simulink model "PubIfDecisionTOS_MDL"  (R2020b)
settings: configuration reference "DspaceConfig" (kept outside this file)
PostLoadFcn:
  | if any(exist('dsrtsu_mdlpostloadfcn', 'file') ~= 0), dsrtsu_mdlpostloadfcn('Execute', bdroot); end
InitFcn:
  | , if any(exist('dsmpb_private', 'file') ~= 0), dsmpb_private('dsmpb_mdlclblib', 'Init', bdroot); end,
undefined symbols (not defined in the file or in its folder): C_TOS_ACCEgoRAxletoFbumplength_m, C_TOS_ACCTargetFront_Flag, C_TOS_AEBJAPedObjDxThre_Val, C_TOS_AEBJAPedObjDyThre_Val, C_TOS_AEBJATargetSize_Val, C_TOS_AEBJAVehObjDxThre_Val, C_TOS_AEBJAVehObjDyThre_Val, C_TOS_AEBJuncPedTargetSize_Val, C_TOS_AEBLatObjDxThre_Val, C_TOS_AEBLatPedDyThre_Val, C_TOS_AEBLatTargetSize_Val, C_TOS_AEBLongTargetInEgoFront_Flag, C_TOS_axAbsGround_Parameter, C_TOS_CameraConfirmedFlag, C_TOS_CNsubjWidth, C_TOS_CurrentLaneCoreMinWidth_Val, C_TOS_CutInProb_Val_Zero, C_TOS_CutOutProb_Val_Zero, C_TOS_D2R_Val, C_TOS_DefaultValueObjectToCenterLine_dy, C_TOS_EgoCarWidth_Val, C_TOS_EgoDxRefPoint_m, C_TOS_EgoRAxletoFbumplength_m, C_TOS_HalfWidthVehicle_Con, C_TOS_HWA_CurrentLaneFlag, C_TOS_HWA_LeftLaneFlag, C_TOS_HWA_MovingDir_Vaild, C_TOS_HWA_MovState_Vaild, C_TOS_HWA_RightLaneFlag, C_TOS_LaneLineCourseErrorFront, C_TOS_LaneLineCourseErrorRear, C_TOS_MotorbikeDefaultWidth_m, C_TOS_NumberOfEffectiveTargets, C_TOS_Obj_Age_Val, C_TOS_Objdx_Constraint_Val, C_TOS_ObjectDefaultWidth_m, C_TOS_ObjInCurrentLane_Val, C_TOS_ObjInCurrentLaneValid, C_TOS_ObjInLeftLaneValid, C_TOS_ObjInRightLaneValid, C_TOS_ObjNotInCurrentLane_Val, C_TOS_ObjNotREElementType, C_TOS_ObjPredictDis_dy_ConstantVal_Zeros, C_TOS_ObjToCenterLine_ConstantVal_Zeros, C_TOS_OFMObjIDInvilad_Val, C_TOS_PIL_LatDisCons_Val_zero, C_TOS_PIL_ObjectCutInFlag_b, C_TOS_PIL_ObjectCutOutFlag_b, C_TOS_PIL_ObjLaneProb_al_Val, C_TOS_PP_ObjFusType_FC_Confirm_b, C_TOS_PP_ObjFusType_FC_FR_Confirm_b, C_TOS_PP_ObjFusType_FR_Confirm_b, C_TOS_RE_80BoolDefault_Val, C_TOS_RE_80Single181Default_Val, C_TOS_RE_80Single255Default_Val, C_TOS_RE_80Uint8Default_Val, C_TOS_RE_D2R, C_TOS_RE_D_180_Val, C_TOS_RE_InvalidObjectID_Val, C_TOS_RE_InvalidTargetChainDir_Val ... (+142)
libraries: simulink x1650, TOS_LIB x361, canfdmsglib x14
(part 47 of 69)

== system PubIfDecisionTOS_MDL/TOS_20201112/TOS_2012080320/TOS/AEB/TOS_AEBJunct_20201208/AEBJunc_Object_Condition1/AEBJA_TargetCondition/TOS_AEBJunc_TargetsCondition/AEBJunc_VehTargetCondition/AEBJunc_VehTargetObjectTypeFlag ==
  ObjectType : Inport
  AEBJunc_VehTarget_ID_K1 : Inport  Port=2
  ObjectID : Inport  Port=3
  AEBJunc_VehTargetObjectTypeAborDly : Subsystem
  Compare To Constant3 : simulink/Logic and Bit Operations/Compare To Constant  relop===  const=OFM_OBJ_TYPE_E.CAR  OutDataTypeStr=boolean
      settings: AttributesFormatString=%<const>
  Compare To Constant4 : simulink/Logic and Bit Operations/Compare To Constant  relop===  const=OFM_OBJ_TYPE_E.TRUCK  OutDataTypeStr=boolean
      settings: AttributesFormatString=%<const>
  Data Type Conversion : DataTypeConversion  OutDataTypeStr=Enum: OFM_OBJ_TYPE_E
  Logical Operator3 : Logic  Operator=OR  AllPortsSameDT=off  OutDataTypeStr=boolean
  AEBJunc_VehTargetObjectTypeFlag : Outport
  wires:
  AEBJunc_VehTargetObjectTypeAborDly/1(TOS_AEBJunc_VehObjectTypeFilt) -> AEBJunc_VehTargetObjectTypeFlag/1
  ObjectID/1 -> AEBJunc_VehTargetObjectTypeAborDly/2(ObjectID)
  AEBJunc_VehTarget_ID_K1/1 -> AEBJunc_VehTargetObjectTypeAborDly/1(AEBJunc_VehTarget_ID_K1)
  Compare To Constant4/1 -> Logical Operator3/2
  Compare To Constant3/1 -> Logical Operator3/1
  Data Type Conversion/1 -> Compare To Constant4/1, Compare To Constant3/1
  ObjectType/1 -> Data Type Conversion/1
  Logical Operator3/1 -> AEBJunc_VehTargetObjectTypeAborDly/3(TOS_AEBJunc_VehObjectType)

== system PubIfDecisionTOS_MDL/TOS_20201112/TOS_2012080320/TOS/AEB/TOS_AEBJunct_20201208/AEBJunc_Object_Condition1/AEBJA_TargetCondition/TOS_AEBJunc_TargetsCondition/AEBJunc_VehTargetCondition/Subsystem ==
  Object_MovingState : Inport
  Compare To Constant1 : simulink/Logic and Bit Operations/Compare To Constant  relop===  const=OFM_OBJ_MOVINGSTATE_E.MOVING  OutDataTypeStr=boolean
      settings: AttributesFormatString=%<const> = 2
  Compare To Constant2 : simulink/Logic and Bit Operations/Compare To Constant  relop===  const=OFM_OBJ_MOVINGSTATE_E.MOVING_SLOWLY  OutDataTypeStr=boolean
      settings: AttributesFormatString=%<const> = 5
  Data Type Conversion : DataTypeConversion  OutDataTypeStr=Enum: OFM_OBJ_MOVINGSTATE_E
  Logical Operator1 : Logic  Operator=OR  AllPortsSameDT=off  OutDataTypeStr=boolean
  TOS_AEBJuncVehTargetMovStateFlg : Outport
  wires:
  Data Type Conversion/1 -> Compare To Constant1/1, Compare To Constant2/1
  Object_MovingState/1 -> Data Type Conversion/1
  Compare To Constant2/1 -> Logical Operator1/2
  Logical Operator1/1 -> TOS_AEBJuncVehTargetMovStateFlg/1
  Compare To Constant1/1 -> Logical Operator1/1

== system PubIfDecisionTOS_MDL/TOS_20201112/TOS_2012080320/TOS/AEB/TOS_AEBJunct_20201208/AEBJunc_Object_Condition1/AEBJA_TargetCondition/TOS_AEBJunc_TargetsCondition/AEBJunc_VehTargetCondition/TOS_AEBJunc_VehTargetMoveDir ==
  Object_Dx : Inport
  PP_ObjMovingDirSignalProcessing : Inport  Port=2
  Object_HeadingAngle : Inport  Port=3
  Object_VX : Inport  Port=4
  Object_VY : Inport  Port=5
  VIE_EgoVelocity : Inport  Port=6
  axvRefMs2 : Inport  Port=7
  Abs{,1..3} (4 alike) : Abs
  Add{,2..4} (4 alike) : Sum
  Add1 : Sum  Inputs=+-
  Compare To Constant : simulink/Logic and Bit Operations/Compare To Constant  relop=<  const=P_TOS_OncomingTarget_VxabsOffset_val  OutDataTypeStr=boolean
      settings: AttributesFormatString=%<const> = -0.7m/s
  Compare To Constant1 : simulink/Logic and Bit Operations/Compare To Constant  relop=>  const=P_TOS_CrossingTargetVyvThre_val  OutDataTypeStr=boolean
      settings: AttributesFormatString=%<const>
  Compare To Constant16 : simulink/Logic and Bit Operations/Compare To Constant  relop=>  const=P_TOS_ObjLatCroYawAngMaxThre_Val  OutDataTypeStr=boolean
      settings: AttributesFormatString=P_TOS_ObjLatCroYawAngMaxThre_Val = 135
  Compare To Constant2 : simulink/Logic and Bit Operations/Compare To Constant  relop===  const=ObjectMovingOrientation_E.OnComingDir  OutDataTypeStr=boolean
      settings: AttributesFormatString=%<const>
  Compare To Constant3 : simulink/Logic and Bit Operations/Compare To Constant  relop=>  const=P_TOS_ObjOncomingYawAngMaxThre_Val  OutDataTypeStr=boolean
      settings: AttributesFormatString=P_TOS_ObjOncomingYawAngMaxThre_Val = 180
  Compare To Constant4 : simulink/Logic and Bit Operations/Compare To Constant  relop=<  const=0  OutDataTypeStr=boolean
  Constant : Constant  Value=C_TOS_StepTime_Val
  Constant1 : Constant  Value=C_TOS_StepTime_Val
  Constant2 : Constant  Value=P_TOS_OncomingVehDxChangeOffset_Val
  Data Type Conversion2 : DataTypeConversion  OutDataTypeStr=Enum: ObjectMovingOrientation_E
  Gain : Gain  Gain=1/2
  Gain1 : Gain  Gain=1/2
  Logical Operator : Logic  Operator=OR  Inputs=4  AllPortsSameDT=off  OutDataTypeStr=boolean
  Logical Operator{1..3,10} (4 alike) : Logic  AllPortsSameDT=off  OutDataTypeStr=boolean
  Math Function : Math  Operator=square  SaturateOnIntegerOverflow=on
  Product : Product
  Product1 : Product
  Relational Operator : RelationalOperator  Operator=>  OutDataTypeStr=boolean  RndMeth=Simplest
  Unit Delay{,1..3} (4 alike) : UnitDelay  InitialCondition=255  SampleTime=-1  HasFrameUpgradeWarning=on
  TOS_AEBJuncVehTargetMovDirFlg : Outport
  wires:
  Logical Operator3/1 -> Logical Operator2/2
  Unit Delay3/1 -> Logical Operator3/2
  Add4/1 -> Relational Operator/2
  Constant2/1 -> Add4/2
  Unit Delay2/1 -> Product/1
  Gain1/1 -> Product1/1
  Add3/1 -> Gain1/1
  Unit Delay1/1 -> Add3/2
  Logical Operator2/1 -> Logical Operator/4
  Relational Operator/1 -> Logical Operator3/1, Unit Delay3/1
  Add2/1 -> Add4/1
  axvRefMs2/1 -> Unit Delay1/1, Add3/1
  Product/1 -> Add2/1
  Gain/1 -> Add2/2
  Product1/1 -> Gain/1
  Math Function/1 -> Product1/2
  Constant1/1 -> Math Function/1
  Constant/1 -> Product/2
  [VIE_EgoVelocity] -> Unit Delay2/1
  Abs3/1 -> Relational Operator/1
  Object_VY/1 -> Abs2/1
  Compare To Constant4/1 -> Logical Operator2/1
  Add1/1 -> Abs3/1, Compare To Constant4/1
  Unit Delay/1 -> Add1/2
  Object_Dx/1 -> Unit Delay/1, Add1/1
  Compare To Constant3/1 -> Logical Operator10/2
  Object_HeadingAngle/1 -> Abs/1
  Compare To Constant2/1 -> Logical Operator/1
  Object_VX/1 -> Add/1
  Compare To Constant16/1 -> Logical Operator10/1
  Logical Operator10/1 -> Logical Operator/2
  Add/1 -> Abs1/1
  Compare To Constant1/1 -> Logical Operator1/2
  Abs/1 -> Compare To Constant3/1, Compare To Constant16/1
  Data Type Conversion2/1 -> Compare To Constant2/1
  Abs1/1 -> Compare To Constant/1
  Compare To Constant/1 -> Logical Operator1/1
  PP_ObjMovingDirSignalProcessing/1 -> Data Type Conversion2/1
  Abs2/1 -> Compare To Constant1/1
  Logical Operator1/1 -> Logical Operator/3
  VIE_EgoVelocity/1 -> Add/2, [VIE_EgoVelocity]
  Logical Operator/1 -> TOS_AEBJuncVehTargetMovDirFlg/1

== system PubIfDecisionTOS_MDL/TOS_20201112/TOS_2012080320/TOS/AEB/TOS_AEBLatCro1105/AEBLat_Object_Condition/AEBLat_TargetCondition/TOS_AEBLat_TargetsDx/AEBLat_TargetObjectTypeFlag/AEBLat_TargetObjectTypeAborDly ==
  AEBLat_Target_ID_K1 : Inport
  ObjectID : Inport  Port=2
  TOS_AEBLat_ObjectType : Inport  Port=3
  Compare To Constant : simulink/Logic and Bit Operations/Compare To Constant  relop=>=  const=1  OutDataTypeStr=boolean
  If : If  IfExpression=u1
  If Action Subsystem : Subsystem  TreatAsAtomicUnit=on
  If Action Subsystem1 : Subsystem  TreatAsAtomicUnit=on
  Merge : Merge
  Subsystem : Subsystem
  Sum of Elements : Sum  Inputs=+
  TOS_AEBLatObjectTypeFilt : Outport
  wires:
  If/1 -> If Action Subsystem1/Action
  TOS_AEBLat_ObjectType/1 -> If Action Subsystem1/1(TOS_AEBLat_ObjectType), If Action Subsystem/1(TOS_AEBLat_ObjectType)
  If/2 -> If Action Subsystem/Action
  AEBLat_Target_ID_K1/1 -> Subsystem/1(ACC_TargetP0_ID_K1)
  ObjectID/1 -> Subsystem/2(ObjectID)
  Subsystem/1(ACC_SameTargetP0) -> Sum of Elements/1
  If Action Subsystem1/1(TOS_AEBLat_ObjectTypeFilt) -> Merge/1
  If Action Subsystem/1(TOS_AEBLat_ObjectTypeFilt) -> Merge/2
  Merge/1 -> TOS_AEBLatObjectTypeFilt/1
  Sum of Elements/1 -> Compare To Constant/1
  Compare To Constant/1 -> If/1

== system PubIfDecisionTOS_MDL/TOS_20201112/TOS_2012080320/TOS/AEB/TOS_AEBLatCro_20201208/AEBLat_Object_Condition/AEBLat_TargetCondition/TOS_AEBLat_TargetsDx/AEBLat_TargetObjectTypeFlag/AEBLat_TargetObjectTypeAborDly ==
  AEBLat_Target_ID_K1 : Inport
  ObjectID : Inport  Port=2
  TOS_AEBLat_ObjectType : Inport  Port=3
  Compare To Constant : simulink/Logic and Bit Operations/Compare To Constant  relop=>=  const=1  OutDataTypeStr=boolean
  If : If  IfExpression=u1
  If Action Subsystem : Subsystem  TreatAsAtomicUnit=on
  If Action Subsystem1 : Subsystem  TreatAsAtomicUnit=on
  Merge : Merge
  Subsystem : Subsystem
  Sum of Elements : Sum  Inputs=+
  TOS_AEBLatObjectTypeFilt : Outport
  wires:
  If/1 -> If Action Subsystem1/Action
  TOS_AEBLat_ObjectType/1 -> If Action Subsystem1/1(TOS_AEBLat_ObjectType), If Action Subsystem/1(TOS_AEBLat_ObjectType)
  If/2 -> If Action Subsystem/Action
  AEBLat_Target_ID_K1/1 -> Subsystem/1(ACC_TargetP0_ID_K1)
  ObjectID/1 -> Subsystem/2(ObjectID)
  Subsystem/1(ACC_SameTargetP0) -> Sum of Elements/1
  If Action Subsystem1/1(TOS_AEBLat_ObjectTypeFilt) -> Merge/1
  If Action Subsystem/1(TOS_AEBLat_ObjectTypeFilt) -> Merge/2
  Merge/1 -> TOS_AEBLatObjectTypeFilt/1
  Sum of Elements/1 -> Compare To Constant/1
  Compare To Constant/1 -> If/1

== system PubIfDecisionTOS_MDL/TOS_20201112/TOS_2012080320/TOS/AEB/TOS_AEBLatCro_20201208/AEBLat_Object_Condition/AEBLat_TargetCondition/TOS_AEBLat_TargetsDx/TOS_AEBLat_TargetMoveDir/AEBLat_TargetMovDirAborDly ==
  AEBLat_Target_ID_K1 : Inport
  ObjectID : Inport  Port=2
  TOS_AEBLat_MovDir_Flag : Inport  Port=3
  Compare To Constant : simulink/Logic and Bit Operations/Compare To Constant  relop=>=  const=1  OutDataTypeStr=boolean
  If : If  IfExpression=u1
  If Action Subsystem : Subsystem  TreatAsAtomicUnit=on
  If Action Subsystem1 : Subsystem  TreatAsAtomicUnit=on
  Merge : Merge
  Subsystem : Subsystem
  Sum of Elements : Sum  Inputs=+
  TOS_AEBLat_MovDirFlag_Delay : Outport
  wires:
  If/1 -> If Action Subsystem1/Action
  TOS_AEBLat_MovDir_Flag/1 -> If Action Subsystem1/1(TOS_AEBLat_MovDir_Flag), If Action Subsystem/1(TOS_AEBLat_MovDir_Flag)
  If/2 -> If Action Subsystem/Action
  AEBLat_Target_ID_K1/1 -> Subsystem/1(ACC_TargetP0_ID_K1)
  ObjectID/1 -> Subsystem/2(ObjectID)
  Subsystem/1(ACC_SameTargetP0) -> Sum of Elements/1
  If Action Subsystem1/1(TOS_AEBLat_MovDirFlag_Delay) -> Merge/1
  If Action Subsystem/1(TOS_AEBLat_MovDirFlag) -> Merge/2
  Merge/1 -> TOS_AEBLat_MovDirFlag_Delay/1
  Sum of Elements/1 -> Compare To Constant/1
  Compare To Constant/1 -> If/1

== system PubIfDecisionTOS_MDL/TOS_20201112/TOS_2012080320/TOS/AEB/TOS_AEBLong/AEBLong_Confirm/AEBLong/AEBLong_TrgConfirm/AEBLongTrgJudg/AEBLong_OverlapRatio ==
  PIL_OverlapRatio : Inport
  Compare To Constant : simulink/Logic and Bit Operations/Compare To Constant  relop=>  const=P_TOS_AEBLong_TargetOverlapThre_Val  OutDataTypeStr=boolean
  AEBLong_OverlapRatioFlag : Outport
  wires:
  Compare To Constant/1 -> AEBLong_OverlapRatioFlag/1
  PIL_OverlapRatio/1 -> Compare To Constant/1

== system PubIfDecisionTOS_MDL/TOS_20201112/TOS_2012080320/TOS/AEB/TOS_AEBLong/AEBLong_Confirm/AEBLong/AEBLong_TrgConfirm/AEBLongTrgJudg/TOS_AEBLong_Dy ==
  Object_DY : Inport
  Object_DX : Inport  Port=2
  <Object_Type> : Inport  Port=3
  Abs{,1..3} (4 alike) : Abs
  Bus Creator : BusCreator  Inputs=3
  Bus Selector : BusSelector  OutputSignals=Object_Type
  Bus Selector1 : BusSelector  OutputSignals=Object_DY
  Bus Selector2 : BusSelector  OutputSignals=Object_DX
  Bus Selector3 : BusSelector  OutputSignals=Object_Type
  Bus Selector4 : BusSelector  OutputSignals=Object_DY
  Bus Selector5 : BusSelector  OutputSignals=Object_DX
  Compare To Constant1 : simulink/Logic and Bit Operations/Compare To Constant  relop===  const=OFM_OBJ_TYPE_E.UNKNOWN_TYPE  OutDataTypeStr=boolean
      settings: AttributesFormatString=OFM_OBJ_TYPE_E.UNKNOWN_TYPE = 1
  Compare To Constant10 : simulink/Logic and Bit Operations/Compare To Constant  relop===  const=OFM_OBJ_TYPE_E.CAR  OutDataTypeStr=boolean
      settings: AttributesFormatString=OFM_OBJ_TYPE_E.CAR = 2
  Compare To Constant2 : simulink/Logic and Bit Operations/Compare To Constant  relop===  const=OFM_OBJ_TYPE_E.MOTORBIKE  OutDataTypeStr=boolean
      settings: AttributesFormatString=OFM_OBJ_TYPE_E.MOTORBIKE = 4
  Compare To Constant3 : simulink/Logic and Bit Operations/Compare To Constant  relop===  const=OFM_OBJ_TYPE_E.PEDESTRIAN  OutDataTypeStr=boolean
      settings: AttributesFormatString=OFM_OBJ_TYPE_E.PEDESTRIAN = 6
  Compare To Constant4 : simulink/Logic and Bit Operations/Compare To Constant  relop===  const=OFM_OBJ_TYPE_E.BICYCLE  OutDataTypeStr=boolean
      settings: AttributesFormatString=OFM_OBJ_TYPE_E.BICYCLE = 5
  Compare To Constant5 : simulink/Logic and Bit Operations/Compare To Constant  relop===  const=OFM_OBJ_TYPE_E.GENERAL_OBJECT  OutDataTypeStr=boolean
      settings: AttributesFormatString=OFM_OBJ_TYPE_E.GENERAL_OBJECT = 7
  Compare To Constant6 : simulink/Logic and Bit Operations/Compare To Constant  relop===  const=OFM_OBJ_TYPE_E.ANIMAL  OutDataTypeStr=boolean
      settings: AttributesFormatString=OFM_OBJ_TYPE_E.ANIMAL = 8
  Compare To Constant7 : simulink/Logic and Bit Operations/Compare To Constant  relop===  const=OFM_OBJ_TYPE_E.INVALID  OutDataTypeStr=boolean
      settings: AttributesFormatString=OFM_OBJ_TYPE_E.INVALID = 0
  Compare To Constant8 : simulink/Logic and Bit Operations/Compare To Constant  relop===  const=OFM_OBJ_TYPE_E.TRUCK  OutDataTypeStr=boolean
      settings: AttributesFormatString=OFM_OBJ_TYPE_E.TRUCK = 3
  Data Type Conversion1 : DataTypeConversion  OutDataTypeStr=Enum: OFM_OBJ_TYPE_E
  Data Type Conversion2 : DataTypeConversion  OutDataTypeStr=Enum: OFM_OBJ_TYPE_E
  Logical Operator : Logic  AllPortsSameDT=off  OutDataTypeStr=boolean
  Logical Operator1 : Logic  Operator=OR  Inputs=7  AllPortsSameDT=off  OutDataTypeStr=boolean
  Logical Operator2 : Logic  AllPortsSameDT=off  OutDataTypeStr=boolean
  Logical Operator3 : Logic  Operator=OR  AllPortsSameDT=off  OutDataTypeStr=boolean
  Logical Operator4 : Logic  Operator=OR  AllPortsSameDT=off  OutDataTypeStr=boolean
  Relational Operator : RelationalOperator  Operator=<=  OutDataTypeStr=boolean  RndMeth=Simplest
  Relational Operator1 : RelationalOperator  Operator=<=  OutDataTypeStr=boolean  RndMeth=Simplest
  data2 : Lookup_n-D  NumberOfTableDimensions=1  BreakpointsForDimension1=[0,40,45,55,60,65,70,95,115,140]  Table=[2.4,2.4,2.4,2.4,3.1,3.1,3.1,3.1,3.3,3.3]  RndMeth=Simplest  InputSameDT=on
  data4 : Lookup_n-D  NumberOfTableDimensions=1  BreakpointsForDimension1=[0,40,45,55,60,65,70,95,115,140]  Table=[1.3,1.4,1.6,1.6,1.9,1.9,1.9,1.9,2.4,2.4]  RndMeth=Simplest  InputSameDT=on
  TOS_AEBLongDy : Outport
  wires:
  Logical Operator4/1 -> TOS_AEBLongDy/1
  Logical Operator2/1 -> Logical Operator4/2
  Logical Operator/1 -> Logical Operator4/1
  Relational Operator1/1 -> Logical Operator2/1
  Abs2/1 -> data2/1
  data2/1 -> Relational Operator1/2
  Abs3/1 -> Relational Operator1/1
  Bus Creator/1 -> Bus Selector1/1, Bus Selector/1, Bus Selector5/1, Bus Selector3/1, Bus Selector4/1, Bus Selector2/1
  Bus Selector3/1 -> Data Type Conversion1/1  "<Object_Type>"
  Compare To Constant10/1 -> Logical Operator3/1
  Bus Selector5/1 -> Abs2/1  "<Object_DX>"
  Bus Selector4/1 -> Abs3/1  "<Object_DY>"
  Data Type Conversion1/1 -> Compare To Constant8/1, Compare To Constant10/1
  Compare To Constant8/1 -> Logical Operator3/2
  Logical Operator3/1 -> Logical Operator2/2
  Logical Operator1/1 -> Logical Operator/2
  Compare To Constant7/1 -> Logical Operator1/7
  Compare To Constant6/1 -> Logical Operator1/6
  Compare To Constant5/1 -> Logical Operator1/5
  Compare To Constant4/1 -> Logical Operator1/4
  Compare To Constant2/1 -> Logical Operator1/3
  Compare To Constant1/1 -> Logical Operator1/2
  Data Type Conversion2/1 -> Compare To Constant3/1, Compare To Constant1/1, Compare To Constant2/1, Compare To Constant4/1, Compare To Constant5/1, Compare To Constant6/1, Compare To Constant7/1
  Bus Selector1/1 -> Abs1/1  "<Object_DY>"
  Bus Selector2/1 -> Abs/1  "<Object_DX>"
  Compare To Constant3/1 -> Logical Operator1/1
  Bus Selector/1 -> Data Type Conversion2/1  "<Object_Type>"
  <Object_Type>/1 -> Bus Creator/3
  Abs1/1 -> Relational Operator/1
  data4/1 -> Relational Operator/2
  Abs/1 -> data4/1
  Relational Operator/1 -> Logical Operator/1
  Object_DY/1 -> Bus Creator/1
  Object_DX/1 -> Bus Creator/2

== system PubIfDecisionTOS_MDL/TOS_20201112/TOS_2012080320/TOS/AEB/TOS_AEBLong/AEBLong_Confirm/AEBLong/AEBLong_TrgConfirm/AEBLongTrgJudg/TOS_AEBLong_ObjFusType ==
  note: 针对选中的运动目标，运动状态突变为静止，改变其运动状态为运动
  object_MovingState : Inport
  PP_ObjFusType_FC_FR_Confirm : Inport  Port=2
  PP_ObjFusType_FR_Confirm : Inport  Port=3
  AEBLong_Target_ID_K1 : Inport  Port=4
  AEBLong_Target_ID_K2 : Inport  Port=5
  AEBLong_Target_MovState_K1 : Inport  Port=6
  AEBLong_Target_MovState_K2 : Inport  Port=7
  ObjectID : Inport  Port=8
  Compare To Constant : simulink/Logic and Bit Operations/Compare To Constant  relop===  const=OFM_OBJ_MOVINGSTATE_E.MOVING  OutDataTypeStr=boolean
      settings: AttributesFormatString=OFM_OBJ_MOVINGSTATE_E.MOVING = 2
  Compare To Constant1 : simulink/Logic and Bit Operations/Compare To Constant  relop===  const=OFM_OBJ_MOVINGSTATE_E.MOVING_SLOWLY  OutDataTypeStr=boolean
      settings: AttributesFormatString=OFM_OBJ_MOVINGSTATE_E.MOVING_SLOWLY = 5
  Compare To Constant2 : simulink/Logic and Bit Operations/Compare To Constant  relop===  const=OFM_OBJ_MOVINGSTATE_E.STOPPED  OutDataTypeStr=boolean
      settings: AttributesFormatString=OFM_OBJ_MOVINGSTATE_E.STOPPED = 4
  Compare To Constant3 : simulink/Logic and Bit Operations/Compare To Constant  relop===  const=OFM_OBJ_MOVINGSTATE_E.STATIONARY  OutDataTypeStr=boolean
      settings: AttributesFormatString=OFM_OBJ_MOVINGSTATE_E.STATIONARY = 3
  Compare To Constant4 : simulink/Logic and Bit Operations/Compare To Constant  relop===  const=OFM_OBJ_MOVINGSTATE_E.UNKNOWN  OutDataTypeStr=boolean
      settings: AttributesFormatString=OFM_OBJ_MOVINGSTATE_E.UNKNOWN = 1
  Compare To Constant5 : simulink/Logic and Bit Operations/Compare To Constant  relop===  const=C_TOS_PP_ObjFusType_FC_FR_Confirm_b  OutDataTypeStr=boolean
      settings: AttributesFormatString=C_TOS_PP_ObjFusType_FC_FR_Confirm_b = 1
  Compare To Constant6 : simulink/Logic and Bit Operations/Compare To Constant  relop===  const=C_TOS_PP_ObjFusType_FR_Confirm_b  OutDataTypeStr=boolean
      settings: AttributesFormatString=C_TOS_PP_ObjFusType_FR_Confirm_b = 1
  Compare To Constant8 : simulink/Logic and Bit Operations/Compare To Constant  relop===  const=1  OutDataTypeStr=boolean
  Data Type Conversion1 : DataTypeConversion  OutDataTypeStr=Enum: OFM_OBJ_MOVINGSTATE_E
  Logical Operator1 : Logic  Operator=OR  AllPortsSameDT=off  OutDataTypeStr=boolean
  Logical Operator2 : Logic  AllPortsSameDT=off  OutDataTypeStr=boolean
  Logical Operator3 : Logic  Operator=OR  Inputs=4  AllPortsSameDT=off  OutDataTypeStr=boolean
  Logical Operator4 : Logic  Operator=OR  AllPortsSameDT=off  OutDataTypeStr=boolean
  Logical Operator5 : Logic  AllPortsSameDT=off  OutDataTypeStr=boolean
  Logical Operator6 : Logic  Operator=OR  AllPortsSameDT=off  OutDataTypeStr=boolean
  Subsystem : Subsystem
  TOS_ACCFusionTypeAborDly : Subsystem
  TOS_AEBLongAEBLongObjFusType : Outport
  wires:
  Compare To Constant6/1 -> Logical Operator1/2
  Compare To Constant5/1 -> [FC_FR_other], Logical Operator1/1
  Logical Operator1/1 -> Logical Operator2/1
  object_MovingState/1 -> Data Type Conversion1/1
  Compare To Constant/1 -> Logical Operator3/1
  Compare To Constant1/1 -> Logical Operator3/2
  Logical Operator3/1 -> Logical Operator2/2
  Compare To Constant2/1 -> Logical Operator3/3
  Compare To Constant3/1 -> Logical Operator4/1
  [FC_FR_other] -> Logical Operator5/1
  Logical Operator4/1 -> Logical Operator5/2
  Logical Operator2/1 -> Logical Operator6/1
  Logical Operator5/1 -> Logical Operator6/2
  Logical Operator6/1 -> TOS_ACCFusionTypeAborDly/3(TOS_ACCFusionType)
  Compare To Constant4/1 -> Logical Operator4/2
  PP_ObjFusType_FC_FR_Confirm/1 -> Compare To Constant5/1
  PP_ObjFusType_FR_Confirm/1 -> Compare To Constant6/1
  Compare To Constant8/1 -> Logical Operator3/4
  Subsystem/1(TOS_ObjMovStateCfm) -> Compare To Constant8/1
  ObjectID/1 -> [ObjectID], Subsystem/6(ObjectID)
  AEBLong_Target_ID_K1/1 -> [AEBLong_Target_ID_K1], Subsystem/2(AEBLong_TargetP0_ID_K1)
  AEBLong_Target_MovState_K2/1 -> Subsystem/5(AEBLong_TargetP0_MovState_K2)
  AEBLong_Target_MovState_K1/1 -> Subsystem/4(AEBLong_TargetP0_MovState_K1)
  AEBLong_Target_ID_K2/1 -> Subsystem/3(AEBLong_TargetP0_ID_K2)
  Data Type Conversion1/1 -> Compare To Constant/1, Compare To Constant3/1, Compare To Constant4/1, Subsystem/1(ObjMovState), Compare To Constant2/1, Compare To Constant1/1
  [ObjectID] -> TOS_ACCFusionTypeAborDly/2(ObjectID)
  [AEBLong_Target_ID_K1] -> TOS_ACCFusionTypeAborDly/1(ACC_TargetP0_ID_K1)
  TOS_ACCFusionTypeAborDly/1(TOS_ACCFusionTypeFilt) -> TOS_AEBLongAEBLongObjFusType/1

== system PubIfDecisionTOS_MDL/TOS_20201112/TOS_2012080320/TOS/AEB/TOS_AEBLong/AEBLong_Confirm/AEBLong/AEBLong_TrgConfirm/AEBLongTrgJudg/TOS_AEBLong_ObstacleProb ==
  note: 参考值：Prob=0.45
  Object_ObstacleProb : Inport
  AEBLong_Target_ID_K1 : Inport  Port=2
  ObjectID : Inport  Port=3
  Compare To Constant : simulink/Logic and Bit Operations/Compare To Constant  relop=>=  const=P_TOS_AEBLongTargetObstacleProbThre_Valu  OutDataTypeStr=boolean
      settings: AttributesFormatString=P_TOS_AEBLongTargetObstacleProbThre_Valu = 0.4
  TOS_ACCObstacleProbAborDly : Subsystem
  TOS_AEBLongObstacleProbFlag : Outport
  wires:
  Compare To Constant/1 -> TOS_ACCObstacleProbAborDly/3(TOS_ACCMovingDir)
  Object_ObstacleProb/1 -> Compare To Constant/1
  ObjectID/1 -> TOS_ACCObstacleProbAborDly/2(ObjectID)
  AEBLong_Target_ID_K1/1 -> TOS_ACCObstacleProbAborDly/1(AEBLong_Target_ID_K1)
  TOS_ACCObstacleProbAborDly/1(TOS_AEBMovingDirFilt) -> TOS_AEBLongObstacleProbFlag/1

== system PubIfDecisionTOS_MDL/TOS_20201112/TOS_2012080320/TOS/AEB/TOS_AEBLong/AEBLong_Confirm/AEBLong/AEBLong_TrgConfirm/AEBLongTrgJudg/TOS_AEBLong_SteerWheelAngConfirm ==
  SteerWheelAng : Inport
  SteerWheelSpd : Inport  Port=2
  Compare To Constant2 : simulink/Logic and Bit Operations/Compare To Constant  relop=<=  const=P_TOS_SteerWheelAngMax_Val  OutDataTypeStr=boolean
      settings: AttributesFormatString=P_TOS_SteerWheelAngMax_Val = 100
  Compare To Constant3 : simulink/Logic and Bit Operations/Compare To Constant  relop=<=  const=P_TOS_SteerWheelSpdMax_Val  OutDataTypeStr=boolean
      settings: AttributesFormatString=P_TOS_SteerWheelSpdMax_Val = 100
  Logical Operator2 : Logic  AllPortsSameDT=off  OutDataTypeStr=boolean
  TOS_AEBLong_SteerWheelAngConfirm : Outport
  wires:
  Logical Operator2/1 -> TOS_AEBLong_SteerWheelAngConfirm/1
  SteerWheelSpd/1 -> Compare To Constant3/1
  SteerWheelAng/1 -> Compare To Constant2/1
  Compare To Constant2/1 -> Logical Operator2/1
  Compare To Constant3/1 -> Logical Operator2/2

== system PubIfDecisionTOS_MDL/TOS_20201112/TOS_2012080320/TOS/AEB/TOS_AEBLong/AEBLong_Confirm/AEBLong/AEBLong_TrgConfirm/AEBLongTrgJudg/TOS_AEBLong_TargetDis ==
  note: 目标的纵向距离约束
      |
      | 本车速度<30km/h时，输出AEB纵向目标距离≤50m
      | 本车速度≥30km/h时，输出AEB纵向目标距离≤85m
  VIE_EgoVelocity : Inport
  Object_Dx : Inport  Port=2
  Compare To Constant : simulink/Logic and Bit Operations/Compare To Constant  relop=<=  const=P_TOS_AEBLongObjSelectCondition_LatSpd_Val  OutDataTypeStr=boolean
      settings: AttributesFormatString=P_TOS_AEBLongObjSelectCondition_LatSpd_Val = 30 km/h
  Compare To Constant1 : simulink/Logic and Bit Operations/Compare To Constant  relop=<=  const=P_TOS_AEBLongObjSelectMaxDis_Val  OutDataTypeStr=boolean
      settings: AttributesFormatString=P_TOS_AEBLongObjSelectMaxDis_Val = 80 m
  Compare To Constant2 : simulink/Logic and Bit Operations/Compare To Constant  relop=>=  const=P_TOS_AEBLongObjSelectMinDis_Val  OutDataTypeStr=boolean
      settings: AttributesFormatString=P_TOS_AEBLongObjSelectMinDis_Val = 0 m
  Constant1 : Constant  Value=C_TOS_SpeedUnitConversionTO_km_h  OutDataTypeStr=single
      settings: AttributesFormatString=C_TOS_SpeedUnitConversionTO_km_h = 3.6
  Constant2 : Constant  Value=P_TOS_AEBLongObjSelectMinDis_Val  OutDataTypeStr=single
      settings: AttributesFormatString=P_TOS_AEBLongObjSelectMinDis_Val = 50 m
  Constant4 : Constant  Value=P_TOS_AEBLongObjSelectMaxDis_Val  OutDataTypeStr=single
      settings: AttributesFormatString=P_TOS_AEBLongObjSelectMaxDis_Val = 85 m
  Logical Operator2 : Logic  AllPortsSameDT=off  OutDataTypeStr=boolean
  Product : Product
  Switch : Switch  Criteria=u2 ~= 0
  Terminator : Terminator
  TOS_TargetDxThreflg : Outport
  wires:
  Switch/1 -> Terminator/1
  Constant2/1 -> Switch/1
  Constant4/1 -> Switch/3
  Compare To Constant/1 -> Switch/2
  Product/1 -> Compare To Constant/1
  Constant1/1 -> Product/2
  VIE_EgoVelocity/1 -> Product/1
  Object_Dx/1 -> Compare To Constant2/1, Compare To Constant1/1
  Logical Operator2/1 -> TOS_TargetDxThreflg/1
  Compare To Constant1/1 -> Logical Operator2/1
  Compare To Constant2/1 -> Logical Operator2/2

== system PubIfDecisionTOS_MDL/TOS_20201112/TOS_2012080320/TOS/AEB/TOS_AEBLong/AEBLong_Confirm/AEBLong/AEBLong_TrgConfirm/AEBLongTrgJudg/TOS_AEBLong_TargetExistProb ==
  Object_ExistProb : Inport
  Compare To Constant : simulink/Logic and Bit Operations/Compare To Constant  relop=>=  const=P_TOS_AEBLongTargetExistProbThre_Valu  OutDataTypeStr=boolean
      settings: AttributesFormatString=P_TOS_AEBLongTargetExistProbThre_Valu = 0.6
  TOS_AEBLongTargetExistProbFlag : Outport
  wires:
  Compare To Constant/1 -> TOS_AEBLongTargetExistProbFlag/1
  Object_ExistProb/1 -> Compare To Constant/1

== system PubIfDecisionTOS_MDL/TOS_20201112/TOS_2012080320/TOS/AEB/TOS_AEBLong/AEBLong_Confirm/AEBLong/AEBLong_TrgConfirm/AEBLongTrgJudg/TOS_AEBLong_TargetInEgoFront ==
  Object_Dx : Inport
  TLJ_TargetInCLValidityflg : Inport  Port=2
  Compare To Constant : simulink/Logic and Bit Operations/Compare To Constant  relop===  const=C_TOS_AEBLongTargetInEgoFront_Flag  OutDataTypeStr=boolean
      settings: AttributesFormatString=C_TOS_AEBLongTargetInEgoFront_Flag = 1
  Compare To Constant1 : simulink/Logic and Bit Operations/Compare To Constant  relop=>=  const=C_TOS_EgoRAxletoFbumplength_m  OutDataTypeStr=boolean
      settings: AttributesFormatString=C_TOS_EgoRAxletoFbumplength_m = 0
  Logical Operator5 : Logic  AllPortsSameDT=off  OutDataTypeStr=boolean
  TOS_TargetInEgoFrontflg : Outport
  wires:
  Compare To Constant/1 -> Logical Operator5/1
  TLJ_TargetInCLValidityflg/1 -> Compare To Constant/1
  Compare To Constant1/1 -> Logical Operator5/2
  Object_Dx/1 -> Compare To Constant1/1
  Logical Operator5/1 -> TOS_TargetInEgoFrontflg/1

== system PubIfDecisionTOS_MDL/TOS_20201112/TOS_2012080320/TOS/AEB/TOS_AEBLong/AEBLong_Confirm/AEBLong/AEBLong_TrgConfirm/AEBLongTrgJudg/TOS_AEBLong_TargetMovingDir ==
  note: 去除横穿目标
  note: 已选中目标，前两个周期为运动，以后为运动，前两个周期为Stopped，以后为Stopped
  object_MovingState : Inport
  PP_ObjMovingDirSignalProcessing : Inport  Port=2
  Object_HeadingAngle : Inport  Port=3
  Object_VX : Inport  Port=4
  Object_VY : Inport  Port=5
  VIE_EgoVelocity : Inport  Port=6
  SteerWheelAngle : Inport  Port=7
  AEBLong_Target_ID_K1 : Inport  Port=8
  AEBLong_Target_ID_K2 : Inport  Port=9
  AEBLong_Target_MovState_K1 : Inport  Port=10
  AEBLong_Target_MovState_K2 : Inport  Port=11
  ObjectID : Inport  Port=12
  Abs{,1..2,5} (4 alike) : Abs
  Add : Sum
  Compare To Constant : simulink/Logic and Bit Operations/Compare To Constant  relop===  const=ObjectMovingOrientation_E.SameDir  OutDataTypeStr=boolean
      settings: AttributesFormatString=ObjectMovingOrientation_E.SameDir = 1
  Compare To Constant1 : simulink/Logic and Bit Operations/Compare To Constant  relop===  const=OFM_OBJ_MOVINGSTATE_E.MOVING  OutDataTypeStr=boolean
      settings: AttributesFormatString=OFM_OBJ_MOVINGSTATE_E.MOVING = 2
  Compare To Constant10 : simulink/Logic and Bit Operations/Compare To Constant  relop=<=  const=P_TOS_ObjLatCroYawAngMaxThre_Val  OutDataTypeStr=boolean
      settings: AttributesFormatString=P_TOS_ObjLatCroYawAngMaxThre_Val = 135
  Compare To Constant11 : simulink/Logic and Bit Operations/Compare To Constant  relop===  const=1  OutDataTypeStr=boolean
  Compare To Constant12 : simulink/Logic and Bit Operations/Compare To Constant  relop=>=  const=P_TOS_ObjInSameDirYawAngMaxThre_Val  OutDataTypeStr=boolean
      settings: AttributesFormatString=P_TOS_ObjInSameDirYawAngMaxThre_Val = 45
  Compare To Constant2 : simulink/Logic and Bit Operations/Compare To Constant  relop=>=  const=P_TOS_ObjInSameDirYawAngMinThre_Val  OutDataTypeStr=boolean
      settings: AttributesFormatString=P_TOS_ObjInSameDirYawAngMinThre_Val = 0
  Compare To Constant3 : simulink/Logic and Bit Operations/Compare To Constant  relop=<=  const=P_TOS_ObjInSameDirYawAngMaxThre_Val  OutDataTypeStr=boolean
      settings: AttributesFormatString=P_TOS_ObjInSameDirYawAngMaxThre_Val = 45
  Compare To Constant4 : simulink/Logic and Bit Operations/Compare To Constant  relop===  const=OFM_OBJ_MOVINGSTATE_E.MOVING_SLOWLY  OutDataTypeStr=boolean
      settings: AttributesFormatString=OFM_OBJ_MOVINGSTATE_E.MOVING_SLOWLY = 5
  Compare To Constant5 : simulink/Logic and Bit Operations/Compare To Constant  relop=<  const=P_TOS_SameDirVyOffset_Val  OutDataTypeStr=boolean
      settings: AttributesFormatString=P_TOS_SameDirVyOffset_Val = 2
  Compare To Constant6 : simulink/Logic and Bit Operations/Compare To Constant  relop===  const=2  OutDataTypeStr=boolean
  Compare To Constant7 : simulink/Logic and Bit Operations/Compare To Constant  relop===  const=OFM_OBJ_MOVINGSTATE_E.STOPPED  OutDataTypeStr=boolean
      settings: AttributesFormatString=OFM_OBJ_MOVINGSTATE_E.STOPPED = 4
  Compare To Constant8 : simulink/Logic and Bit Operations/Compare To Constant  relop===  const=ObjectMovingOrientation_E.Crossing  OutDataTypeStr=boolean
      settings: AttributesFormatString=ObjectMovingOrientation_E.Crossing = 3
  Compare To Constant9 : simulink/Logic and Bit Operations/Compare To Constant  relop=>=  const=P_TOS_LongVyThre_Val  OutDataTypeStr=boolean
      settings: AttributesFormatString=P_TOS_LongVyThre_Val = 2
  Constant1 : Constant  Value=P_TOS_SameDirVxvOffset_Val
      settings: AttributesFormatString=P_TOS_AEBLong_SameDirVxvOffset_Val = 1
  Constant2 : Constant  OutDataTypeStr=boolean
  Constant3 : Constant  Value=0  OutDataTypeStr=boolean
  Constant4 : Constant  OutDataTypeStr=boolean
  Data Type Conversion1 : DataTypeConversion  OutDataTypeStr=Enum: ObjectMovingOrientation_E
  Data Type Conversion2 : DataTypeConversion  OutDataTypeStr=Enum: OFM_OBJ_MOVINGSTATE_E
  Logical Operator : Logic  AllPortsSameDT=off  OutDataTypeStr=boolean
  Logical Operator{1,4..6} (4 alike) : Logic  Operator=OR  AllPortsSameDT=off  OutDataTypeStr=boolean
  Logical Operator2 : Logic  Operator=OR  Inputs=3  AllPortsSameDT=off  OutDataTypeStr=boolean
  Logical Operator3 : Logic  AllPortsSameDT=off  OutDataTypeStr=boolean
  Logical Operator8 : Logic  AllPortsSameDT=off  OutDataTypeStr=boolean
  ObjMovingDirSignalProcessing1 : Subsystem  Commented=on
  Obj_MovingDir : Subsystem  Commented=on
  Relational Operator : RelationalOperator  Operator=<  OutDataTypeStr=boolean  RndMeth=Simplest
  Subsystem : Subsystem
  Switch : Switch  Criteria=u2 ~= 0
  Switch1 : Switch  Criteria=u2 ~= 0
  Switch2 : Switch  Criteria=u2 ~= 0
  TOS_ACCMovingDirAborDly : Subsystem
  Terminator : Terminator
  Terminator1 : Terminator
  Terminator2 : Terminator
  TOS_AEBLongMovingDirFlg : Outport
  wires:
  PP_ObjMovingDirSignalProcessing/1 -> Data Type Conversion1/1
  Logical Operator1/1 -> Switch/1
  Data Type Conversion1/1 -> [PP_ObjMovingDirSignalProcessing], Compare To Constant/1
  Compare To Constant2/1 -> Logical Operator3/1
  Compare To Constant3/1 -> Logical Operator3/2
  Abs/1 -> [Object_HeadingAngle], Compare To Constant3/1, Compare To Constant2/1
  Object_HeadingAngle/1 -> Abs/1
  Compare To Constant/1 -> Logical Operator1/1
  Logical Operator3/1 -> Terminator1/1
  object_MovingState/1 -> Data Type Conversion2/1
  Compare To Constant4/1 -> Logical Operator2/2
  Compare To Constant1/1 -> Logical Operator2/1
  Logical Operator2/1 -> Switch/2
  Switch/1 -> TOS_ACCMovingDirAborDly/3(TOS_ACCMovingDir)
  VIE_EgoVelocity/1 -> Relational Operator/2
  Add/1 -> Relational Operator/1
  Abs1/1 -> Add/1
  Constant1/1 -> Add/2
  Object_VX/1 -> Abs1/1
  Relational Operator/1 -> Logical Operator/1
  Object_VY/1 -> [Object_VY], Abs2/1
  Abs2/1 -> Compare To Constant5/1
  Compare To Constant5/1 -> Logical Operator/2
  Logical Operator/1 -> Logical Operator1/2
  Constant3/1 -> Switch2/1
  Abs5/1 -> Compare To Constant9/1
  Logical Operator8/1 -> Logical Operator4/2
  Compare To Constant10/1 -> Logical Operator8/2
  Compare To Constant9/1 -> Switch2/2, Logical Operator6/2
  Compare To Constant12/1 -> Logical Operator8/1
  [Object_HeadingAngle] -> Compare To Constant10/1, Compare To Constant12/1
  [PP_ObjMovingDirSignalProcessing] -> Compare To Constant8/1
  Compare To Constant8/1 -> Logical Operator4/1
  [Object_VY] -> Abs5/1
  Constant4/1 -> Switch2/3
  SteerWheelAngle/1 -> Terminator/1
  [AEBLong_Target_ID_K1] -> TOS_ACCMovingDirAborDly/1(AEBLong_Target_ID_K1)
  [ObjectID] -> TOS_ACCMovingDirAborDly/2(ObjectID)
  TOS_ACCMovingDirAborDly/1(TOS_AEBMovingDirFilt) -> TOS_AEBLongMovingDirFlg/1
  Compare To Constant11/1 -> Logical Operator2/3
  Compare To Constant6/1 -> Logical Operator5/1
  AEBLong_Target_ID_K1/1 -> [AEBLong_Target_ID_K1], Subsystem/2(AEBLong_Target_ID_K1)
  Compare To Constant7/1 -> Logical Operator5/2
  AEBLong_Target_MovState_K1/1 -> Subsystem/4(AEBLong_Target_MovState_K1)
  AEBLong_Target_ID_K2/1 -> Subsystem/3(AEBLong_Target_ID_K2)
  Data Type Conversion2/1 -> Compare To Constant7/1, Subsystem/1(ObjMovState), Compare To Constant4/1, Compare To Constant1/1
  AEBLong_Target_MovState_K2/1 -> Subsystem/5(AEBLong_Target_MovState_K2)
  Subsystem/1(TOS_ObjMovStateCfm) -> Compare To Constant11/1, Compare To Constant6/1
  ObjectID/1 -> [ObjectID], Subsystem/6(ObjectID)
  Logical Operator5/1 -> Switch1/2
  Switch1/1 -> Switch/3
  Switch2/1 -> Switch1/3
  Constant2/1 -> Switch1/1
  Logical Operator4/1 -> Logical Operator6/1
  Logical Operator6/1 -> Terminator2/1

== system PubIfDecisionTOS_MDL/TOS_20201112/TOS_2012080320/TOS/AEB/TOS_AEBLong/AEBLong_Confirm/AEBLong/AEBLong_TrgConfirm/AEBLongTrgJudg/TOS_AEB_Stockade ==
  note: fun1; 静态 / 雷达探测目标 / 做距离限制，约束栅栏
  PP_ObjFusType_FR_Confirm : Inport
  object_MovingState : Inport  Port=2
  Object_DX : Inport  Port=3
  ObjectToCenterLine_dy : Inport  Port=4
  Object_Type : Inport  Port=5
  Abs : Abs
  Compare To Constant1 : simulink/Logic and Bit Operations/Compare To Constant  relop===  const=OFM_OBJ_MOVINGSTATE_E.INVALID  OutDataTypeStr=boolean
      settings: AttributesFormatString=OFM_OBJ_MOVINGSTATE_E.INVALID = 0
  Compare To Constant2 : simulink/Logic and Bit Operations/Compare To Constant  relop===  const=OFM_OBJ_TYPE_E.UNKNOWN_TYPE  OutDataTypeStr=boolean
      settings: AttributesFormatString=OFM_OBJ_TYPE_E.UNKNOWN_TYPE = 1
  Compare To Constant3 : simulink/Logic and Bit Operations/Compare To Constant  relop===  const=OFM_OBJ_TYPE_E.INVALID  OutDataTypeStr=boolean
      settings: AttributesFormatString=OFM_OBJ_TYPE_E.INVALID = 0
  Compare To Constant4 : simulink/Logic and Bit Operations/Compare To Constant  relop===  const=C_TOS_PP_ObjFusType_FR_Confirm_b  OutDataTypeStr=boolean
      settings: AttributesFormatString=C_TOS_PP_ObjFusType_FR_Confirm_b = 1
  Compare To Constant6 : simulink/Logic and Bit Operations/Compare To Constant  relop===  const=OFM_OBJ_MOVINGSTATE_E.STATIONARY  OutDataTypeStr=boolean
      settings: AttributesFormatString=OFM_OBJ_MOVINGSTATE_E.STATIONARY = 3
  Compare To Constant7 : simulink/Logic and Bit Operations/Compare To Constant  relop===  const=OFM_OBJ_MOVINGSTATE_E.UNKNOWN  OutDataTypeStr=boolean
      settings: AttributesFormatString=OFM_OBJ_MOVINGSTATE_E.UNKNOWN = 1
  Constant : Constant  Value=0  OutDataTypeStr=boolean
  Constant1 : Constant  OutDataTypeStr=boolean
  Data Type Conversion1 : DataTypeConversion  OutDataTypeStr=Enum: OFM_OBJ_MOVINGSTATE_E
  Data Type Conversion2 : DataTypeConversion  OutDataTypeStr=Enum: OFM_OBJ_TYPE_E
  LaneWidthWeight : Lookup_n-D  NumberOfTableDimensions=1  BreakpointsForDimension1=[0,50,60,70,80,100]  Table=[1.2,1.2,0.9,0.7,0.5,0.5]  RndMeth=Simplest  InputSameDT=on
  Logical Operator1 : Logic  Operator=OR  AllPortsSameDT=off  OutDataTypeStr=boolean
  Logical Operator2 : Logic  Operator=OR  AllPortsSameDT=off  OutDataTypeStr=boolean
  Logical Operator8 : Logic  Inputs=3  AllPortsSameDT=off  OutDataTypeStr=boolean
  Relational Operator : RelationalOperator  Operator=<=  OutDataTypeStr=boolean  RndMeth=Nearest
  Switch : Switch  Criteria=u2 ~= 0
  Switch1 : Switch  Criteria=u2 ~= 0
  TOS_AEB_Stockade : Outport
  wires:
  Compare To Constant4/1 -> Logical Operator8/1
  PP_ObjFusType_FR_Confirm/1 -> Compare To Constant4/1
  object_MovingState/1 -> Data Type Conversion1/1
  Compare To Constant6/1 -> Logical Operator2/1
  Data Type Conversion1/1 -> Compare To Constant1/1, Compare To Constant7/1, Compare To Constant6/1
  Logical Operator8/1 -> Switch/2
  Switch1/1 -> Switch/3
  LaneWidthWeight/1 -> Relational Operator/2  "factor"
  Object_DX/1 -> LaneWidthWeight/1
  ObjectToCenterLine_dy/1 -> Abs/1  "ObjectToCenterLine_dy"
  Relational Operator/1 -> Switch/1  "Lat_dy"
  Abs/1 -> Relational Operator/1
  Data Type Conversion2/1 -> Compare To Constant2/1, Compare To Constant3/1
  Object_Type/1 -> Data Type Conversion2/1
  Compare To Constant2/1 -> Logical Operator8/3
  Constant/1 -> Switch1/1
  Constant1/1 -> Switch1/3
  Logical Operator1/1 -> Switch1/2
  Compare To Constant7/1 -> Logical Operator2/2
  Logical Operator2/1 -> Logical Operator8/2
  Compare To Constant1/1 -> Logical Operator1/1
  Compare To Constant3/1 -> Logical Operator1/2
  Switch/1 -> TOS_AEB_Stockade/1
